simulink library "HORTISIM"  (R2021a)
settings: Solver=VariableStepAuto  StartTime=0.0  StopTime=10.0  RelTol=1e-3
undefined symbols (not defined in the file or in its folder): crop_params, heat_ic, heat_p, p_climate, params_fruit, scr_p, substrate_params, tp_tilapia, win_p, x0_climate, x0_crop, x0_fruit, x0_substrate, x0_tank_tilapia
libraries: $bdroot x10
(part 2 of 4)

== system HORTISIM/Climate/Models/Climate Model/Gases Exchange ==
  Indoor Temperature : Inport
  Transpiration Heat : Inport  Port=2
  Ventilation Rate : Inport  Port=3
  Condensation : Inport  Port=4
  In Bus Element : Inport  Port=5  PortName=EC  Element=Temp
  In Bus Element1 : Inport  Port=5  PortName=EC  Element=HR
  Carbon Consumption : Inport  Port=6
  CO2 Pump : Inport  Port=7
  Carbon Dynamics : Subsystem
      settings: PortSchema="{\"entries\":[{\"content\":{\"sides\":[{\"content\":{\"connectorIds\":[\"In1\",\"In2\",\"In3\"]},\"type\":\"ConnectorPlacement.EquallySpacedRectSide\",\"uuid\":\"ce6da3e3-21f1-4394-8848-c3b9ed37cfe4\"},{\"content\":{\"connectorIds\":[\"Out1\",\"Out2\"],\"side\":\"RIGHT\"},\"type\":\"ConnectorPlacement.EquallySpacedRectSide\",\"uuid\":\"ff9d1dc7-ad1d-4f02-8424-55a857bc099f\"},{\"content\":{\"connectorIds\":[\"In4\",\"In5\"],\"side\":\"TOP\"},\"type\":\"ConnectorPlacement.EquallySpacedRectSide\",\"uuid\":\"728a06d8-4ce2-49f0-80dc-b6302b266d7a\"}]},\"type\":\"ConnectorPlacement.EquallySpacedConnector\",\"uuid\":\"a07ea8b7-add0-4d37-8d5e-856da5f5b640\"}],\"packageUris\":[\"http://schema.mathworks.com/mf0/Connector/R2020b\"],\"version\":\"1.0\"}"
  Compute Mid Variables : Subsystem
      settings: PortSchema="{\"entries\":[{\"content\":{\"sides\":[{\"content\":{\"connectorIds\":[\"In1\",\"In2\"]},\"type\":\"ConnectorPlacement.EquallySpacedRectSide\",\"uuid\":\"c9e251e2-f19d-4856-b15c-3b9f1eb64f83\"},{\"content\":{\"connectorIds\":[\"Out1\"],\"side\":\"RIGHT\"},\"type\":\"ConnectorPlacement.EquallySpacedRectSide\",\"uuid\":\"10734817-c937-42fb-8ae5-9505620c6f0f\"},{\"content\":{\"connectorIds\":[],\"side\":\"TOP\"},\"type\":\"ConnectorPlacement.EquallySpacedRectSide\",\"uuid\":\"8c056440-d8bf-4ff4-85aa-0f6a5eb7f23f\"},{\"content\":{\"connectorIds\":[\"In3\"],\"side\":\"BOTTOM\"},\"type\":\"ConnectorPlacement.EquallySpacedRectSide\",\"uuid\":\"fc2511c5-58d6-455e-9438-4abf6bda86a2\"}]},\"type\":\"ConnectorPlacement.EquallySpacedConnector\",\"uuid\":\"13e72cfa-9d8f-4756-adac-f24fb0238c2a\"}],\"packageUris\":[\"http://schema.mathworks.com/mf0/Connector/R2020b\"],\"version\":\"1.0\"}"
  Gain1 : Gain  Gain=24*3600
  Integrator1 : Integrator  InitialCondition=x0.G0  AbsoluteTolerance=1e-5
  Vector Concatenate : Concatenate
  Water Dynamics : Subsystem
      settings: PortSchema="{\"entries\":[{\"content\":{\"sides\":[{\"content\":{\"connectorIds\":[\"In1\",\"In2\",\"In3\"]},\"type\":\"ConnectorPlacement.EquallySpacedRectSide\",\"uuid\":\"ce6da3e3-21f1-4394-8848-c3b9ed37cfe4\"},{\"content\":{\"connectorIds\":[\"Out1\"],\"side\":\"RIGHT\"},\"type\":\"ConnectorPlacement.EquallySpacedRectSide\",\"uuid\":\"ff9d1dc7-ad1d-4f02-8424-55a857bc099f\"},{\"content\":{\"connectorIds\":[\"In4\"],\"side\":\"TOP\"},\"type\":\"ConnectorPlacement.EquallySpacedRectSide\",\"uuid\":\"728a06d8-4ce2-49f0-80dc-b6302b266d7a\"},{\"content\":{\"connectorIds\":[\"In5\",\"In6\"],\"side\":\"BOTTOM\"},\"type\":\"ConnectorPlacement.EquallySpacedRectSide\",\"uuid\":\"cc1d9c53-b6c6-41b0-b878-c109c9de6d5f\"}]},\"type\":\"ConnectorPlacement.EquallySpacedConnector\",\"uuid\":\"a07ea8b7-add0-4d37-8d5e-856da5f5b640\"}],\"packageUris\":[\"http://schema.mathworks.com/mf0/Connector/R2020b\"],\"version\":\"1.0\"}"
  " Gas" : Outport
  wires:
  Gain1/1 -> Integrator1/1
  Vector Concatenate/1 -> Gain1/1
  Integrator1/1 -> Compute Mid Variables/1(Gas_Conc)
  Transpiration Heat/1 -> Water Dynamics/2(Latent Heat)
  Water Dynamics/1(dC_w_dt) -> Vector Concatenate/1
  Carbon Consumption/1 -> Carbon Dynamics/1(CarbonC)
  Carbon Dynamics/1(dC_c_dt) -> Vector Concatenate/2
  Ventilation Rate/1 -> Carbon Dynamics/5(Ventilation Rate), Water Dynamics/6(Ventilation Rate)
  Indoor Temperature/1 -> Compute Mid Variables/2(Indoor Temperature)
  Compute Mid Variables/1(Gas) -> Water Dynamics/1(GasComp), Carbon Dynamics/3(GasComp), " Gas"/1
  Condensation/1 -> Water Dynamics/3(Condensation)
  CO2 Pump/1 -> Carbon Dynamics/2(MC_cc_i)
  In Bus Element/1 -> Carbon Dynamics/4(Te), Water Dynamics/5(Te)
  In Bus Element1/1 -> Water Dynamics/4(He)
  Carbon Dynamics/2(C_ce) -> Compute Mid Variables/3(C_ce)

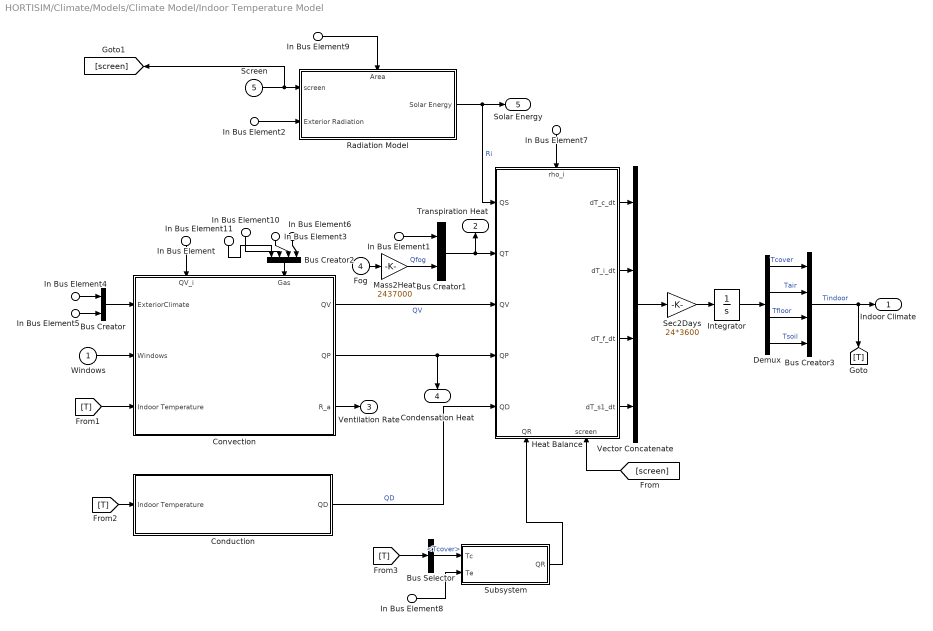
== system HORTISIM/Climate/Models/Climate Model/Indoor Temperature Model ==
  Windows : Inport
  In Bus Element2 : Inport  Port=2  PortName=EC  Element=Rad
  In Bus Element4 : Inport  Port=2  PortName=EC  Element=Temp
  In Bus Element8 : Inport  Port=2  PortName=EC  Element=Temp
  In Bus Element5 : Inport  Port=2  PortName=EC  Element=Wind
  In Bus Element : Inport  Port=3  PortName=External  Element=QV
  In Bus Element1 : Inport  Port=3  PortName=External  Element=QT
  In Bus Element9 : Inport  Port=3  PortName=External  Element=A
  Fog : Inport  Port=4
  Screen : Inport  Port=5
  In Bus Element3 : Inport  Port=6  PortName=Gas  Element=C_w
  In Bus Element6 : Inport  Port=6  PortName=Gas  Element=rho_i
  In Bus Element7 : Inport  Port=6  PortName=Gas  Element=rho_i
  In Bus Element10 : Inport  Port=6  PortName=Gas  Element=C_w_sat_T_c
  In Bus Element11 : Inport  Port=6  PortName=Gas  Element=C_w_sat_T_f
  Bus Creator : BusCreator  Inputs=2
  Bus Creator1 : BusCreator  Inputs=2
  Bus Creator2 : BusCreator  Inputs=4
  Bus Creator3 : BusCreator  Inputs=4
  Bus Selector : BusSelector  OutputSignals=Tcover
  Conduction : Subsystem
  Convection : Subsystem
      settings: PortSchema="{\"entries\":[{\"content\":{\"sides\":[{\"content\":{\"connectorIds\":[\"In1\",\"In2\",\"In3\"]},\"type\":\"ConnectorPlacement.EquallySpacedRectSide\",\"uuid\":\"3a7e199a-659d-4634-89e1-ef85cb7ed502\"},{\"content\":{\"connectorIds\":[\"Out1\",\"Out2\",\"Out3\"],\"side\":\"RIGHT\"},\"type\":\"ConnectorPlacement.EquallySpacedRectSide\",\"uuid\":\"10ed7806-8be5-4e88-a0ca-6abfb5c9ab8d\"},{\"content\":{\"connectorIds\":[\"In4\",\"In5\"],\"side\":\"TOP\"},\"type\":\"ConnectorPlacement.EquallySpacedRectSide\",\"uuid\":\"907defe4-ff8f-4a74-ba27-620529c27b74\"},{\"content\":{\"connectorIds\":[],\"side\":\"BOTTOM\"},\"type\":\"ConnectorPlacement.EquallySpacedRectSide\",\"uuid\":\"397bdb42-e8ee-4be9-8569-3130f6cbf999\"}]},\"type\":\"ConnectorPlacement.EquallySpacedConnector\",\"uuid\":\"f437f85f-61b6-4f41-a544-29e333cf1086\"}],\"packageUris\":[\"http://schema.mathworks.com/mf0/Connector/R2020b\"],\"version\":\"1.0\"}"
  Demux : Demux
  Heat Balance : Subsystem
      settings: PortSchema="{\"entries\":[{\"content\":{\"sides\":[{\"content\":{\"connectorIds\":[\"In1\",\"In2\",\"In3\",\"In4\",\"In5\"]},\"type\":\"ConnectorPlacement.EquallySpacedRectSide\",\"uuid\":\"ccfbb954-e9e7-4841-9dc1-a760315eb250\"},{\"content\":{\"connectorIds\":[\"Out1\",\"Out2\",\"Out3\",\"Out4\"],\"side\":\"RIGHT\"},\"type\":\"ConnectorPlacement.EquallySpacedRectSide\",\"uuid\":\"e9754eb2-54ce-43cf-bf33-7cf2f1345c42\"},{\"content\":{\"connectorIds\":[\"In6\"],\"side\":\"TOP\"},\"type\":\"ConnectorPlacement.EquallySpacedRectSide\",\"uuid\":\"6ccd5de1-b6bb-47c5-ac6c-9382e354fee6\"},{\"content\":{\"connectorIds\":[\"In7\",\"In8\"],\"side\":\"BOTTOM\"},\"type\":\"ConnectorPlacement.EquallySpacedRectSide\",\"uuid\":\"dba41702-708c-4231-8998-8d54661f4881\"}]},\"type\":\"ConnectorPlacement.EquallySpacedConnector\",\"uuid\":\"31920c9d-5e0f-4503-9ddd-ce99d792a3e0\"}],\"packageUris\":[\"http://schema.mathworks.com/mf0/Connector/R2020b\"],\"version\":\"1.0\"}"
  Integrator : Integrator  InitialCondition=x0.T0  AbsoluteTolerance=0.01
  Mass2Heat : Gain  Gain=2437000
  Radiation Model : Subsystem
      settings: PortSchema="{\"entries\":[{\"content\":{\"sides\":[{\"content\":{\"connectorIds\":[\"In1\",\"In2\"]},\"type\":\"ConnectorPlacement.EquallySpacedRectSide\",\"uuid\":\"cb5a2538-07d5-409a-bc47-ac7157db0ef4\"},{\"content\":{\"connectorIds\":[\"Out1\"],\"side\":\"RIGHT\"},\"type\":\"ConnectorPlacement.EquallySpacedRectSide\",\"uuid\":\"7dfe2e6f-8ee6-45c0-8502-080571e1b483\"},{\"content\":{\"connectorIds\":[\"In3\"],\"side\":\"TOP\"},\"type\":\"ConnectorPlacement.EquallySpacedRectSide\",\"uuid\":\"52df64bb-9cf1-44e4-8c24-fa6c372d73f1\"}]},\"type\":\"ConnectorPlacement.EquallySpacedConnector\",\"uuid\":\"b803895f-b114-4368-b273-36a7794022b5\"}],\"packageUris\":[\"http://schema.mathworks.com/mf0/Connector/R2020b\"],\"version\":\"1.0\"}"
  Sec2Days : Gain  Gain=24*3600
  Subsystem : Subsystem
  Vector Concatenate : Concatenate  NumInputs=4
  Indoor Climate : Outport
  Transpiration Heat : Outport  Port=2
  Ventilation Rate : Outport  Port=3
  Condensation Heat : Outport  Port=4
  Solar Energy : Outport  Port=5
  wires:
  [screen] -> Heat Balance/8(screen)
  Vector Concatenate/1 -> Sec2Days/1
  Sec2Days/1 -> Integrator/1
  Convection/3(R_a) -> Ventilation Rate/1
  Convection/1(QV) -> Heat Balance/3(QV)  "QV"
  Conduction/1(QD) -> Heat Balance/5(QD)  "QD"
  Heat Balance/2(dT_i_dt) -> Vector Concatenate/2
  Heat Balance/3(dT_f_dt) -> Vector Concatenate/3
  Heat Balance/4(dT_s1_dt) -> Vector Concatenate/4
  Heat Balance/1(dT_c_dt) -> Vector Concatenate/1
  [T] -> Convection/3(Indoor Temperature)
  [T] -> Conduction/1(Indoor Temperature)
  In Bus Element7/1 -> Heat Balance/6(rho_i)
  Convection/2(QP) -> Condensation Heat/1, Heat Balance/4(QP)
  Windows/1 -> Convection/2(Windows)
  In Bus Element2/1 -> Radiation Model/2(Exterior Radiation)
  Radiation Model/1("Solar Energy  ") -> Solar Energy/1, Heat Balance/1(QS)  "Ri"
  Bus Creator/1 -> Convection/1(ExteriorClimate)
  Screen/1 -> Radiation Model/1(screen), [screen]
  In Bus Element4/1 -> Bus Creator/1
  In Bus Element5/1 -> Bus Creator/2
  Fog/1 -> Mass2Heat/1
  Mass2Heat/1 -> Bus Creator1/2  "Qfog"
  In Bus Element1/1 -> Bus Creator1/1
  Bus Creator1/1 -> Heat Balance/2(QT), Transpiration Heat/1
  Bus Creator2/1 -> Convection/5(Gas)
  In Bus Element3/1 -> Bus Creator2/3
  In Bus Element6/1 -> Bus Creator2/4
  In Bus Element/1 -> Convection/4(QV_i)
  Bus Creator3/1 -> [T], Indoor Climate/1  "Tindoor"
  Demux/4 -> Bus Creator3/4  "Tsoil"
  Demux/3 -> Bus Creator3/3  "Tfloor"
  Demux/2 -> Bus Creator3/2  "Tair"
  Demux/1 -> Bus Creator3/1  "Tcover"
  Integrator/1 -> Demux/1
  In Bus Element8/1 -> Subsystem/2(Te)
  [T] -> Bus Selector/1
  Bus Selector/1 -> Subsystem/1(Tc)  "<Tcover>"
  Subsystem/1(QR) -> Heat Balance/7(QR)
  In Bus Element9/1 -> Radiation Model/3(Area)
  In Bus Element10/1 -> Bus Creator2/2
  In Bus Element11/1 -> Bus Creator2/1

== system HORTISIM/Climate/Models/Climate Model/Subsystem ==
  Gas : Inport
  Bus Creator3 : BusCreator  Inputs=4
  Bus Selector : BusSelector  OutputSignals=C_w,rho_i,C_w_sat_T_c,C_w_sat_T_f
  Out1 : Outport
  wires:
  Bus Selector/3 -> Bus Creator3/3  "<C_w_sat_T_c>"
  Bus Creator3/1 -> Out1/1
  Bus Selector/1 -> Bus Creator3/1  "<C_w>"
  Bus Selector/2 -> Bus Creator3/2  "<rho_i>"
  Bus Selector/4 -> Bus Creator3/4  "<C_w_sat_T_f>"
  Gas/1 -> Bus Selector/1

== system HORTISIM/Horticulture/Controls/Ferrtirrigation Controler/Irrigation Controler ==
  note: $kg\{H_2O\}/(s\cdot m^2)$
  " " : Gain  Gain=5.6e-3
  Clock2 : Clock
  Constant1 : Constant  Value=24
  Gain4 : Gain  Gain=24
  If : If  IfExpression=(u1 > 6)&(u1<7)
  If Action Subsystem : Subsystem  TreatAsAtomicUnit=on
  If Action Subsystem1 : Subsystem  TreatAsAtomicUnit=on
  Merge : Merge
  Mod : Math  Operator=mod  SaturateOnIntegerOverflow=on
  Irrigation : Outport
  wires:
  " "/1 -> Irrigation/1
  Constant1/1 -> Mod/2
  Clock2/1 -> Gain4/1
  Gain4/1 -> Mod/1
  Mod/1 -> If/1, If Action Subsystem/1(In1)
  If/1 -> If Action Subsystem/Action
  If/2 -> If Action Subsystem1/Action
  If Action Subsystem/1(Out1) -> Merge/1
  If Action Subsystem1/1(Out1) -> Merge/2
  Merge/1 -> " "/1

== system HORTISIM/Horticulture/Models/Crop Grow/Air Convection ==
  QS_v_VIS : Inport
  QT_v_i : Inport  Port=2
  T_i : Inport  Port=3
  <LAI> : Inport  Port=4
  " Temperature" : MATLAB Function  TreatAsAtomicUnit=on
  Bus Creator : BusCreator  Inputs=5
  Constant : Constant  Value=params.A_v
  Gain1 : Gain  Gain=24*3600
  Minus : Sum  Inputs=+-
  Subsystem : Subsystem
      settings: PortSchema="{\"entries\":[{\"content\":{\"sides\":[{\"content\":{\"connectorIds\":[\"In1\",\"In2\"]},\"type\":\"ConnectorPlacement.EquallySpacedRectSide\",\"uuid\":\"4a223777-4148-4e71-aff8-25d93471e208\"},{\"content\":{\"connectorIds\":[\"Out1\",\"Out2\"],\"side\":\"RIGHT\"},\"type\":\"ConnectorPlacement.EquallySpacedRectSide\",\"uuid\":\"f67a472e-d82a-4194-8a1d-cf4d17d79652\"},{\"content\":{\"connectorIds\":[],\"side\":\"TOP\"},\"type\":\"ConnectorPlacement.EquallySpacedRectSide\",\"uuid\":\"dc13fded-a670-4e66-896d-6b985aeea447\"},{\"content\":{\"connectorIds\":[\"In3\"],\"side\":\"BOTTOM\"},\"type\":\"ConnectorPlacement.EquallySpacedRectSide\",\"uuid\":\"546dc1d6-9e48-4e4a-b9dc-c8e8ff8af02b\"}]},\"type\":\"ConnectorPlacement.EquallySpacedConnector\",\"uuid\":\"dd1fea49-cd8b-49b4-879c-c05a742382b3\"}],\"packageUris\":[\"http://schema.mathworks.com/mf0/Connector/R2020b\"],\"version\":\"1.0\"}"
  Tv : Integrator  InitialCondition=x0.Tv  AbsoluteTolerance=0.01
  Tv_mean : Integrator  InitialCondition=x0.Tv  AbsoluteTolerance=1e-3
  surface density [kg/m^2] : Constant  Value=1.326
  HV : Outport
  HeatVars : Outport  Port=2
  wires:
  Gain1/1 -> Tv/1
  " Temperature"/1(dT_v_dt) -> Gain1/1
  surface density [kg/m^2]/1 -> " Temperature"/6(msd_v)
  Constant/1 -> " Temperature"/4(A_v)
  <LAI>/1 -> Subsystem/2(LAI), " Temperature"/5(LAI)
  Subsystem/2(HV) -> HV/1
  T_i/1 -> Subsystem/1(T_i)
  Tv_mean/1 -> [Tv_mu], Minus/2  "Tv_mean"
  Minus/1 -> Tv_mean/1
  Tv/1 -> [Tv], Minus/1, Subsystem/3(T_v)  "Tv"
  Subsystem/1(QV_v_i) -> [QV_v_i], " Temperature"/3(QV_v_i)  "QV"
  QS_v_VIS/1 -> [QS_i]  "QS"
  QT_v_i/1 -> [QT_v_i], " Temperature"/2(QT_v_i)  "QT"
  [Tv] -> Bus Creator/1  "Tveg"
  [Tv_mu] -> Bus Creator/2  "TvegMean"
  [QV_v_i] -> Bus Creator/3
  [QT_v_i] -> Bus Creator/4
  [QS_i] -> Bus Creator/5
  Bus Creator/1 -> HeatVars/1

== system HORTISIM/Horticulture/Models/Crop Grow/Crop Growth ==
  Gas : Inport
  QS_v_VIS : Inport  Port=2
  MC_leaf_prune : Inport  Port=3
  harvest : Inport  Port=4
  RTU : Inport  Port=5
  CropBus : Inport  Port=6
  Temperature : Inport  Port=7
  Bus Creator : BusCreator  Inputs=5
  Gain{1..4} (4 alike) : Gain  Gain=24*3600
  Growth model : Subsystem
      settings: PortSchema="{\"entries\":[{\"content\":{\"sides\":[{\"content\":{\"connectorIds\":[\"In1\",\"In2\",\"In3\",\"In4\",\"In5\"]},\"type\":\"ConnectorPlacement.EquallySpacedRectSide\",\"uuid\":\"524d3e03-5719-41db-bf49-dcf5dd5869ab\"},{\"content\":{\"connectorIds\":[\"Out1\",\"Out2\",\"Out3\",\"Out4\",\"Out5\"],\"side\":\"RIGHT\"},\"type\":\"ConnectorPlacement.EquallySpacedRectSide\",\"uuid\":\"b6ee0c40-6a76-4355-a893-3d13d29f29ea\"},{\"content\":{\"connectorIds\":[\"In6\",\"Out6\"],\"side\":\"TOP\"},\"type\":\"ConnectorPlacement.EquallySpacedRectSide\",\"uuid\":\"3cb45a24-0889-4a9a-ac04-e1ca208b77ae\"}]},\"type\":\"ConnectorPlacement.EquallySpacedConnector\",\"uuid\":\"fab17374-053c-4d8a-b11b-d7cd69978ad8\"}],\"packageUris\":[\"http://schema.mathworks.com/mf0/Connector/R2020b\"],\"version\":\"1.0\"}"
  Integrator1 : Integrator  InitialCondition=x0.N  AbsoluteTolerance=1e-4
  Integrator2 : Integrator  InitialCondition=x0.C  AbsoluteTolerance=1e-4
  Integrator3 : Integrator  InitialCondition=x0.R  AbsoluteTolerance=1e-9
  Integrator4 : Integrator  InitialCondition=x0.Tsum
  Subsystem : Subsystem
  Subsystem1 : Subsystem
  Subsystem2 : Subsystem
      settings: PortSchema="{\"entries\":[{\"content\":{\"sides\":[{\"content\":{\"connectorIds\":[\"In1\"]},\"type\":\"ConnectorPlacement.EquallySpacedRectSide\",\"uuid\":\"1f0226fa-6d14-4434-a5d5-098a94c6aa33\"},{\"content\":{\"connectorIds\":[\"Out1\"],\"side\":\"RIGHT\"},\"type\":\"ConnectorPlacement.EquallySpacedRectSide\",\"uuid\":\"12e08114-9d71-45f9-bd21-e03815fbba92\"},{\"content\":{\"connectorIds\":[],\"side\":\"TOP\"},\"type\":\"ConnectorPlacement.EquallySpacedRectSide\",\"uuid\":\"f70b570c-09d2-427a-8272-34c6eabee9a4\"},{\"content\":{\"connectorIds\":[\"In2\"],\"side\":\"BOTTOM\"},\"type\":\"ConnectorPlacement.EquallySpacedRectSide\",\"uuid\":\"db0772f6-92fe-46fe-85e5-ff48d92542ad\"}]},\"type\":\"ConnectorPlacement.EquallySpacedConnector\",\"uuid\":\"23ce1bc9-4d09-4c56-8e1c-5e49b0ef0462\"}],\"packageUris\":[\"http://schema.mathworks.com/mf0/Connector/R2020b\"],\"version\":\"1.0\"}"
  "Carbon Comp   " : Outport
  Crop : Outport  Port=2
  wires:
  Bus Creator/1 -> Crop/1  "Crop"
  Growth model/6("Carbon Comp   ") -> "Carbon Comp   "/1
  MC_leaf_prune/1 -> Growth model/3(MC_leaf_prune)
  Integrator4/1 -> Bus Creator/4  "Tsum"
  Growth model/3(dRdt) -> Gain3/1
  Gas/1 -> Growth model/1(Gas)
  Gain3/1 -> Integrator3/1
  Gain4/1 -> Integrator4/1
  Growth model/4(dT_vsum_dt) -> Gain4/1
  Growth model/2(dCdt) -> Gain2/1
  QS_v_VIS/1 -> Growth model/2(QS_v_VIS)
  Gain2/1 -> Integrator2/1
  CropBus/1 -> Growth model/4(Crop)
  Temperature/1 -> Growth model/5(Temperature)
  Growth model/5(MC_gro) -> Bus Creator/5  "MC_gro"
  Subsystem/1(Out1) -> Bus Creator/2  "Carbon"
  Integrator2/1 -> Subsystem/1(In1)  "Carbon"
  Integrator3/1 -> Subsystem1/1(In1)  "Relative"
  Subsystem1/1(Out1) -> Bus Creator/3  "Relative"
  Gain1/1 -> Integrator1/1
  RTU/1 -> Gain1/1  "Nuptake"
  Integrator1/1 -> Subsystem2/1(M)  "Nutrients"
  Subsystem2/1(Out1) -> Bus Creator/1  "Nutrients"
  Growth model/1(dN/dt) -> Subsystem2/2(ND)  "Ndemand"
  harvest/1 -> Growth model/6(harvest)

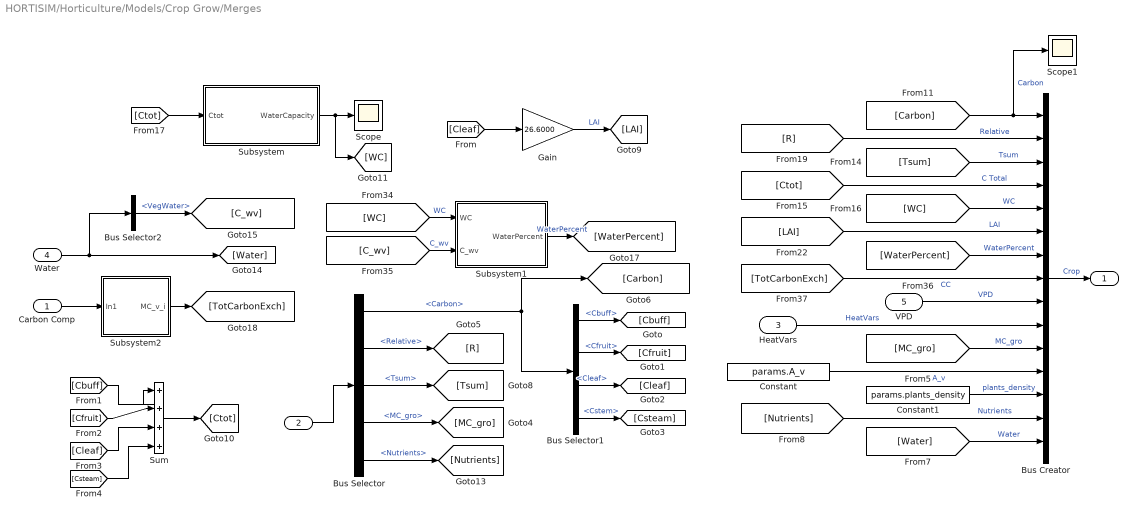
== system HORTISIM/Horticulture/Models/Crop Grow/Merges ==
  "Carbon Comp   " : Inport
  " " : Inport  Port=2
  HeatVars : Inport  Port=3
  Water : Inport  Port=4
  VPD : Inport  Port=5
  Bus Creator : BusCreator  Inputs=15
  Bus Selector : BusSelector  OutputSignals=Carbon,Relative,Tsum,MC_gro,Nutrients
  Bus Selector1 : BusSelector  OutputSignals=Cbuff,Cfruit,Cleaf,Cstem
  Bus Selector2 : BusSelector  OutputSignals=WaterState.VegWater
  Constant : Constant  Value=params.A_v
  Constant1 : Constant  Value=params.plants_density
  Gain : Gain  Gain=26.6000
  Scope : Scope
  Scope1 : Scope
  Subsystem : Subsystem
  Subsystem1 : Subsystem
  Subsystem2 : Subsystem
  Sum : Sum  Inputs=|++++
  "    " : Outport
  wires:
  [Cleaf] -> Gain/1
  Gain/1 -> [LAI]  "LAI"
  Subsystem/1(WaterCapacity) -> [WC], Scope/1
  [Ctot] -> Subsystem/1(Ctot)
  [Cbuff] -> Sum/1
  [Cfruit] -> Sum/2
  [Cleaf] -> Sum/3
  Sum/1 -> [Ctot]
  Bus Selector/1 -> Bus Selector1/1, [Carbon]  "<Carbon>"
  Water/1 -> Bus Selector2/1, [Water]
  [Tsum] -> Bus Creator/3  "Tsum"
  [LAI] -> Bus Creator/6  "LAI"
  [R] -> Bus Creator/2  "Relative"
  " "/1 -> Bus Selector/1
  Bus Selector1/1 -> [Cbuff]  "<Cbuff>"
  Bus Selector1/3 -> [Cleaf]  "<Cleaf>"
  Bus Creator/1 -> "    "/1  "Crop"
  Bus Selector1/4 -> [Csteam]  "<Cstem>"
  [WC] -> Subsystem1/1(WC)  "WC"
  Subsystem1/1(WaterPercent) -> [WaterPercent]  "WaterPercent"
  [TotCarbonExch] -> Bus Creator/8  "CC"
  VPD/1 -> Bus Creator/9  "VPD"
  [WC] -> Bus Creator/5  "WC"
  Bus Selector/4 -> [MC_gro]  "<MC_gro>"
  [MC_gro] -> Bus Creator/11  "MC_gro"
  HeatVars/1 -> Bus Creator/10  "HeatVars"
  [Csteam] -> Sum/4
  Constant/1 -> Bus Creator/12  "A_v"
  [WaterPercent] -> Bus Creator/7  "WaterPercent"
  [Water] -> Bus Creator/15  "Water"
  [Carbon] -> Scope1/1, Bus Creator/1  "Carbon"
  Bus Selector/3 -> [Tsum]  "<Tsum>"
  "Carbon Comp   "/1 -> Subsystem2/1(In1)
  Bus Selector1/2 -> [Cfruit]  "<Cfruit>"
  Bus Selector/2 -> [R]  "<Relative>"
  Bus Selector2/1 -> [C_wv]  "<VegWater>"
  [C_wv] -> Subsystem1/2(C_wv)  "C_wv"
  Subsystem2/1(MC_v_i) -> [TotCarbonExch]
  [Ctot] -> Bus Creator/4  "C Total"
  Constant1/1 -> Bus Creator/13  "plants_density"
  Bus Selector/5 -> [Nutrients]  "<Nutrients>"
  [Nutrients] -> Bus Creator/14  "Nutrients"

== system HORTISIM/Horticulture/Models/Crop Grow/Subsystem ==
  In1 : Inport
  In2 : Inport  Port=2
  In3 : Inport  Port=3
  Bus Selector : BusSelector  OutputSignals=LAI
  Constant1 : Constant  Value=params.A_v
  Gain : Gain  Gain=2
  Product1 : Product  Inputs=3
  Scope : Scope
  Scope1 : Scope
  Subsystem : Subsystem
  Subsystem1 : Subsystem
  Sum : Sum  Inputs=|++
  Sum1 : Sum  Inputs=|++
  Out1 : Outport
  wires:
  In2/1 -> Sum1/2
  Sum1/1 -> Product1/3
  In1/1 -> Sum1/1
  Constant1/1 -> Product1/2
  In3/1 -> Bus Selector/1
  Subsystem/1(Out1) -> Scope/1, [a_v_fVIS]
  Bus Selector/1 -> Subsystem1/1(<LAI>), Subsystem/1(<LAI>)  "<LAI>"
  Subsystem1/1(Out1) -> [a_v_rVIS]
  [a_v_rVIS] -> Sum/1
  [a_v_fVIS] -> Sum/2
  Sum/1 -> Scope1/1, Product1/1
  Product1/1 -> Gain/1
  Gain/1 -> Out1/1

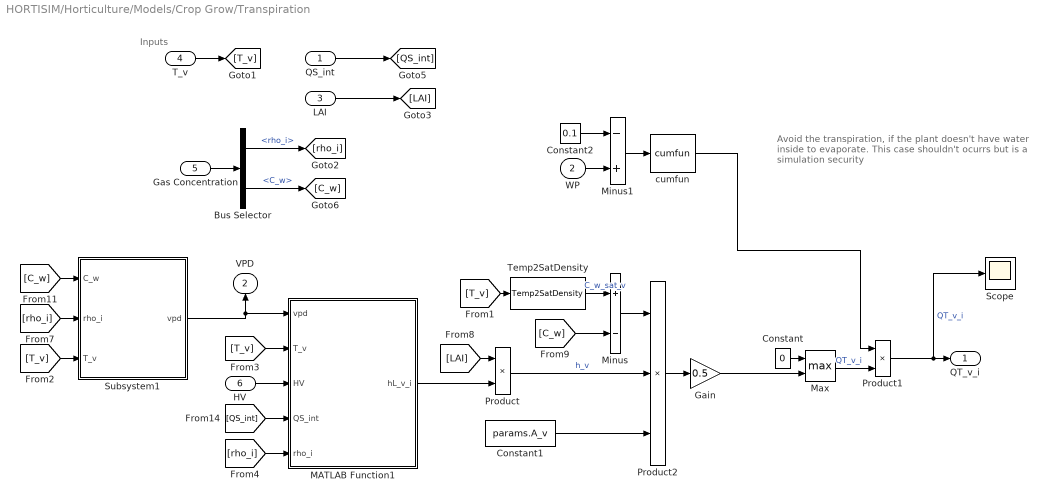
== system HORTISIM/Horticulture/Models/Crop Grow/Transpiration ==
  note: Avoid the transpiration, if the plant
      |  doesn't have water inside to evaporate.
      | This case shouldn't ocurrs but is a simulation security
  note: Inputs
  QS_int : Inport
  WP : Inport  Port=2
  LAI : Inport  Port=3
  T_v : Inport  Port=4
  Gas Concentration : Inport  Port=5
  HV : Inport  Port=6
  Bus Selector : BusSelector  OutputSignals=rho_i,C_w
  Constant : Constant  Value=0
  Constant1 : Constant  Value=params.A_v
  Constant2 : Constant  Value=0.1
  Gain : Gain  Gain=0.5
  MATLAB Function1 : MATLAB Function  TreatAsAtomicUnit=on
  Max : MinMax  Function=max  Inputs=2
  Minus : Sum  Inputs=+-
  Minus1 : Sum  Inputs=-+
  Product : Product
  Product1 : Product
  Product2 : Product  Inputs=3
  Scope : Scope
  Subsystem1 : Subsystem
  Temp2SatDensity : $bdroot/Other  Functions/Temp2SatDensity  SystemSampleTime=-1  VariantActivationTime=update diagram  Latency=0  AutoFrameSizeCalculation=off
  cumfun : $bdroot/Other  Functions/cumfun  SystemSampleTime=-1  VariantActivationTime=update diagram  Latency=0  AutoFrameSizeCalculation=off
  QT_v_i : Outport
  VPD : Outport  Port=2
  wires:
  Gain/1 -> Max/2
  Max/1 -> Product1/2  "QT_v_i"
  Constant/1 -> Max/1
  Product1/1 -> Scope/1, QT_v_i/1  "QT_v_i"
  Product2/1 -> Gain/1
  Constant1/1 -> Product2/3
  Product/1 -> Product2/2  "h_v"
  Minus/1 -> Product2/1
  [C_w] -> Minus/2
  T_v/1 -> [T_v]
  QS_int/1 -> [QS_int]
  Gas Concentration/1 -> Bus Selector/1
  Bus Selector/1 -> [rho_i]  "<rho_i>"
  Bus Selector/2 -> [C_w]  "<C_w>"
  [T_v] -> Temp2SatDensity/1
  Temp2SatDensity/1 -> Minus/1  "C_w_sat_v"
  [C_w] -> Subsystem1/1(C_w)
  [rho_i] -> Subsystem1/2(rho_i)
  [T_v] -> Subsystem1/3(T_v)
  LAI/1 -> [LAI]
  [LAI] -> Product/1
  MATLAB Function1/1(hL_v_i) -> Product/2
  [QS_int] -> MATLAB Function1/4(QS_int)
  HV/1 -> MATLAB Function1/3(HV)
  Subsystem1/1(vpd) -> VPD/1, MATLAB Function1/1(vpd)
  [T_v] -> MATLAB Function1/2(T_v)
  [rho_i] -> MATLAB Function1/5(rho_i)
  WP/1 -> Minus1/2
  Constant2/1 -> Minus1/1
  cumfun/1 -> Product1/1
  Minus1/1 -> cumfun/1

== system HORTISIM/Horticulture/Models/Crop Grow/Water Balance ==
  note: $kg\{H_2O\}/(s\cdot m^2)$
  note: $kg\{H_2O\}/m^2$
  note: $kg\{H_2O\}/(s\cdot m^2)$
  Crop : Inport
  <QT_v_i> : Inport  Port=2
  RWU : Inport  Port=3
  Bus Selector : BusSelector  OutputSignals=WaterPercent,WC,A_v
  Divide : Product  Inputs=*//
  H_fg : Constant  Value=2437000
  Subsystem : Subsystem
  Subsystem1 : Subsystem
  Out Bus Element : Outport  PortName=WaterFlows  Element=WaterDemand
  Out Bus Element1 : Outport  PortName=WaterFlows  Element=WaterUptake
  Out Bus Element3 : Outport  PortName=WaterFlows  Element=MW_QT
  Out Bus Element6 : Outport  Port=2  PortName=WaterState  Element=VegWater
  wires:
  Divide/1 -> [MW_QT], Subsystem/2(Evapotranspiration)  "Evapotranspiration"
  <QT_v_i>/1 -> Divide/1
  H_fg/1 -> Divide/2
  Crop/1 -> Bus Selector/1
  [RWU] -> Out Bus Element1/1  "Real Water Uptake"
  [DemandWater] -> Out Bus Element/1
  Bus Selector/3 -> Divide/3  "<A_v>"
  Bus Selector/1 -> Subsystem1/1(<WaterPercent>)  "<WaterPercent>"
  Bus Selector/2 -> Subsystem1/2(<WC>)  "<WC>"
  Subsystem1/1(Out1) -> [DemandWater]
  RWU/1 -> [RWU], Subsystem/1(Real Water Uptake)  "Real Water Uptake"
  Subsystem/1(C_wv) -> Out Bus Element6/1
  [MW_QT] -> Out Bus Element3/1

== system HORTISIM/Horticulture/Models/Substrate Bag/Nutrient Balance ==
  Irrigation : Inport
  NutrientDemand : Inport  Port=2
  Water : Inport  Port=3
  Bus Creator : BusCreator  Inputs=3  OutDataTypeStr=Bus: FLOW  NonVirtualBus=on
  Bus Selector1 : BusSelector  OutputSignals=X,f,T
  Bus Selector3 : BusSelector  OutputSignals=Water,SusWater.VT,drainge
  Demux : Demux  Outputs=8
  Gain1 : Gain  Gain=24*3600
  Integrator : Integrator  InitialCondition=x0.N
  Minus : Sum  Inputs=-+--
  Product : Product
  Product2 : Product
  Product3 : Product
  Scope : Scope
  Subsystem : Subsystem
  Subsystem1 : Subsystem
  Vector Concatenate : Concatenate  NumInputs=8
  Drainge : Outport
  Mass In Sustrate : Outport  Port=2
  RealNutrientUptake : Outport  Port=3
  wires:
  Irrigation/1 -> Bus Selector1/1  "Irrigation"
  Bus Selector1/1 -> Product/1  "<X>"
  Bus Selector1/2 -> Product/2  "<f>"
  Product/1 -> Demux/1
  Integrator/1 -> Scope/1, Subsystem/2(Mass), Mass In Sustrate/1, Subsystem1/2(Content)
  Product2/1 -> Minus/4
  Bus Selector1/3 -> [T]  "<T>"
  [T] -> Bus Creator/2  "T"
  [D] -> Bus Creator/1  "f"
  Bus Creator/1 -> Drainge/1
  Subsystem/1(X) -> Product3/2, Product2/1, Bus Creator/3
  Vector Concatenate/1 -> Minus/2
  Minus/1 -> Gain1/1
  Gain1/1 -> Integrator/1
  NutrientDemand/1 -> Subsystem1/1(Demand)
  Subsystem1/1(RealNutrientUptake) -> Minus/1, RealNutrientUptake/1
  Water/1 -> Bus Selector3/1
  Bus Selector3/1 -> [WPT]  "<Water>"
  Bus Selector3/2 -> [SW]  "<VT>"
  Bus Selector3/3 -> [D]  "<drainge>"
  [D] -> Product2/2
  [SW] -> Subsystem/1(V)
  [WPT] -> Product3/1
  Product3/1 -> Minus/3
  Demux/8 -> Vector Concatenate/8  "TSS"
  Demux/7 -> Vector Concatenate/7  "O2"
  Demux/6 -> Vector Concatenate/6  "S"
  Demux/5 -> Vector Concatenate/5  "P"
  Demux/4 -> Vector Concatenate/4  "Mg"
  Demux/3 -> Vector Concatenate/3  "Ca"
  Demux/2 -> Vector Concatenate/2  "K"
  Demux/1 -> Vector Concatenate/1  "N"

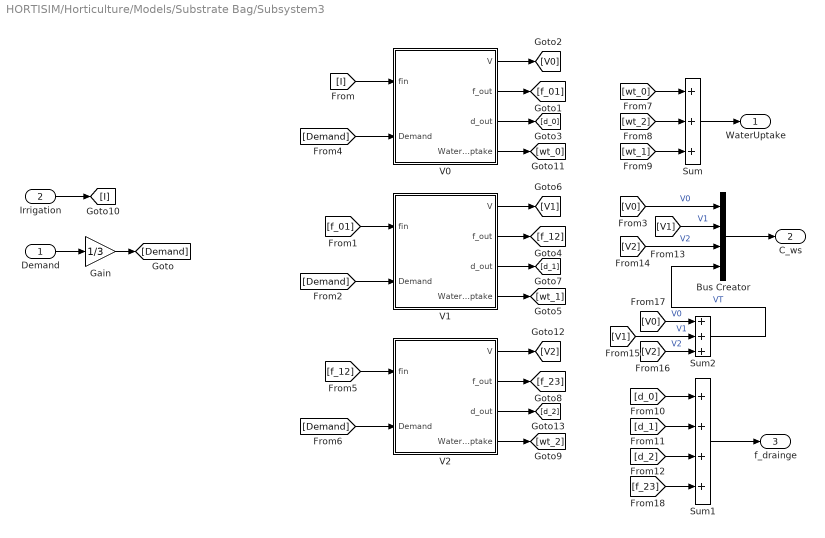
== system HORTISIM/Horticulture/Models/Substrate Bag/Subsystem3 ==
  Demand : Inport
  Irrigation : Inport  Port=2
  Bus Creator : BusCreator  Inputs=4
  Gain : Gain  Gain=1/3
  Sum : Sum  Inputs=+++
  Sum1 : Sum  Inputs=++++
  Sum2 : Sum  Inputs=+++
  V0 : Subsystem
  V1 : Subsystem
  V2 : Subsystem
  WaterUptake : Outport
  C_ws : Outport  Port=2
  f_drainge : Outport  Port=3
  wires:
  [I] -> V0/1(fin)
  V0/1(V) -> [V0]
  V0/2(f_out) -> [f_01]
  V0/3(d_out) -> [d_0]
  Irrigation/1 -> [I]
  Sum1/1 -> f_drainge/1
  Demand/1 -> Gain/1
  Gain/1 -> [Demand]
  [Demand] -> V0/2(Demand)
  V0/4(WaterUptake) -> [wt_0]
  V1/3(d_out) -> [d_1]
  V1/4(WaterUptake) -> [wt_1]
  V1/2(f_out) -> [f_12]
  [Demand] -> V1/2(Demand)
  V1/1(V) -> [V1]
  [f_12] -> V2/1(fin)
  V2/3(d_out) -> [d_2]
  V2/4(WaterUptake) -> [wt_2]
  V2/2(f_out) -> [f_23]
  [Demand] -> V2/2(Demand)
  V2/1(V) -> [V2]
  [f_01] -> V1/1(fin)
  [wt_0] -> Sum/1
  [wt_2] -> Sum/2
  [wt_1] -> Sum/3
  Sum/1 -> WaterUptake/1
  [d_2] -> Sum1/3
  [d_1] -> Sum1/2
  [d_0] -> Sum1/1
  [V0] -> Bus Creator/1  "V0"
  [V1] -> Bus Creator/2  "V1"
  [V2] -> Bus Creator/3  "V2"
  Bus Creator/1 -> C_ws/1
  [V0] -> Sum2/1  "V0"
  [V1] -> Sum2/2  "V1"
  [V2] -> Sum2/3  "V2"
  Sum2/1 -> Bus Creator/4  "VT"
  [f_23] -> Sum1/4

== system HORTISIM/Aquaculture/Models/Tank Model/Heat Balances/Convection Air 2 Water Tanl Surface ==
  T_i : Inport
  A_t : Inport  Port=2
  T_w : Inport  Port=3
  d_t : Inport  Port=4
  wind_speed : Inport  Port=5
  Divide : Product  Inputs=*/
  Gr : Subsystem
  Gr2vG : Subsystem
  Minus : Sum  Inputs=-+
  Product : Product  Inputs=4
  Re : Subsystem
  Re2vR : Subsystem
  Subsystem : Subsystem
  "thermal conductivity of air [W/m/K] " : Constant  Value=0.0250
  QV_i_w : Outport
  wires:
  T_i/1 -> [T_i]
  T_w/1 -> [T_w]
  A_t/1 -> [A_t]
  d_t/1 -> [d_t]
  wind_speed/1 -> [ws]
  [ws] -> Re/2(wind_speed)
  [d_t] -> Re/1(d_w)
  [T_w] -> Gr/3(T_w)
  [T_i] -> Gr/2(T_air)
  [d_t] -> Gr/1(d)
  Gr/1(Gr) -> Gr2vG/1(Gr)
  Re/1(Re) -> Re2vR/1(Re)
  [A_t] -> Divide/1
  [d_t] -> Divide/2
  Subsystem/1(nu) -> Product/3
  Divide/1 -> Product/2
  "thermal conductivity of air [W/m/K] "/1 -> Product/1
  [T_w] -> Minus/1
  [T_i] -> Minus/2
  Minus/1 -> Product/4
  Product/1 -> QV_i_w/1
  Gr2vG/1(Out1) -> Subsystem/1(In1)
  Gr2vG/2(Out2) -> Subsystem/2(In2)
  Re2vR/1(Out1) -> Subsystem/3(In3)
  Re2vR/2(Out2) -> Subsystem/4(In4)

== system HORTISIM/Aquaculture/Models/Tank Model/Heat Balances/Convection Air 2 Water Tanl Surface1 ==
  T_w : Inport
  A_t : Inport  Port=2
  T_wall : Inport  Port=3
  d_t : Inport  Port=4
  Divide : Product  Inputs=*/
  Minus : Sum  Inputs=+-
  Product : Product  Inputs=3
  "thermal conductivity of air [W/m/K] " : Constant  Value=0.6
  QV_i_w : Outport
  wires:
  T_w/1 -> Minus/2
  T_wall/1 -> Minus/1
  A_t/1 -> Divide/1
  d_t/1 -> Divide/2
  Divide/1 -> Product/2
  "thermal conductivity of air [W/m/K] "/1 -> Product/1
  Minus/1 -> Product/3
  Product/1 -> QV_i_w/1

== system HORTISIM/Aquaculture/Models/Tank Model/Heat Balances/Energy Balance ==
  QV_i_W : Inport
  V : Inport  Port=2
  QA : Inport  Port=3
  QT : Inport  Port=4
  QV_wall_water : Inport  Port=5
  Divide : Product  Inputs=*/
  Integrator1 : Integrator  InitialCondition=x0.T
  J/(kg.K) : Constant  Value=4192
  Product : Product  Inputs=3
  Scope : Scope  NumInputPorts=4
  Sum1 : Sum  Inputs=+-++
  kg/m^3 : Constant  Value=997
  seconds to days1 : Gain  Gain=(3600*24)
  Out1 : Outport
  wires:
  QA/1 -> Sum1/4, Scope/4
  Integrator1/1 -> Out1/1
  Product/1 -> Divide/2  "J/K"
  Sum1/1 -> Divide/1
  seconds to days1/1 -> Integrator1/1
  J/(kg.K)/1 -> Product/2
  kg/m^3/1 -> Product/3
  QV_i_W/1 -> Sum1/3, Scope/3
  Divide/1 -> seconds to days1/1
  V/1 -> Product/1
  QT/1 -> Sum1/2, Scope/2
  QV_wall_water/1 -> Sum1/1, Scope/1

== system HORTISIM/Aquaculture/Models/Tank Model/Heat Balances/Transpiration ==
  Air Speed : Inport
  Xh : Inport  Port=2
  Tw : Inport  Port=3
  p_a : Inport  Port=4
  Constant : Constant  Value=0
  Constant1 : Constant  Value=25
  Constant2 : Constant  Value=params.S
  Divide : Product  Inputs=*/
  Gain : Gain  Gain=19
  Gain1 : Gain  Gain=1/3600
  Mass2Heat [J/kg] : Gain  Gain=2437000
  Max : MinMax  Function=max  Inputs=2
  Minus1 : Sum  Inputs=+-
  Product : Product
  Product1 : Product
  Ratio of Humidity Sat : Subsystem
  Scope : Scope  NumInputPorts=3
  Sum1 : Sum  Inputs=|++
  Water Density [kg/m^3] : Constant  Value=997
  QT : Outport
  Evaporation : Outport  Port=2
  wires:
  Max/1 -> Mass2Heat [J/kg]/1, Divide/1
  Constant/1 -> Max/2
  Divide/1 -> Evaporation/1
  Mass2Heat [J/kg]/1 -> QT/1  "Qfog"
  Water Density [kg/m^3]/1 -> Divide/2
  Product1/1 -> Max/1  "MW_evaporation [kg/s]"
  Product/1 -> Gain1/1
  Constant1/1 -> Sum1/2
  Sum1/1 -> Product/1
  Constant2/1 -> Product/2
  Gain1/1 -> Product1/1
  Air Speed/1 -> Gain/1
  Xh/1 -> Scope/3, Minus1/2
  Gain/1 -> Sum1/1
  Minus1/1 -> Scope/1, Product1/2
  Tw/1 -> Ratio of Humidity Sat/1(T)
  p_a/1 -> Ratio of Humidity Sat/2(p_a)
  Ratio of Humidity Sat/1(Out1) -> Minus1/1, Scope/2  "Xh_sat"

== system HORTISIM/Aquaculture/Models/Tank Model/Subsystem/For Each Subsystem ==
  In1 : Inport  Partition=on  PartitionDimension=1  PartitionWidth=1  PartitionOffset=0
  In2 : Inport  Port=2
  For Each : ForEach  DisableCoverage=on
  Product : Product
  Out1 : Outport  ConcatenationDimension=2
  wires:
  In1/1 -> Product/1
  In2/1 -> Product/2
  Product/1 -> Out1/1

== system HORTISIM/Aquaculture/Models/Tank Model/Subsystem/Subsystem1 ==
  Fio : Inport
  X : Inport  Port=2
  T : Inport  Port=3
  Constant : Constant  Value=0
  For Each Subsystem : Subsystem  TreatAsAtomicUnit=on
  For Each Subsystem1 : Subsystem  TreatAsAtomicUnit=on
  Max : MinMax  Function=max  Inputs=2
  Minus : Sum  Inputs=+-
  Product : Product
  Sum of Elements : Sum  Inputs=+
  Sum of Elements1 : Sum  Inputs=+  CollapseMode=Specified dimension  CollapseDim=2
  Transpose : Math  Operator=transpose  SaturateOnIntegerOverflow=on
  density and specify heat of water : Gain  Gain=997*4186
  fT : Outport
  MS : Outport  Port=2
  QA : Outport  Port=3
  wires:
  Constant/1 -> Max/1
  For Each Subsystem/3(T) -> Minus/1
  Max/1 -> Product/1
  density and specify heat of water/1 -> QA/1
  Minus/1 -> Product/2
  Product/1 -> density and specify heat of water/1
  T/1 -> Minus/2
  Fio/1 -> For Each Subsystem/1(Fin)
  For Each Subsystem/1(fs) -> Sum of Elements/1, Max/2, Transpose/1
  Sum of Elements/1 -> fT/1
  For Each Subsystem/2(Xs) -> For Each Subsystem1/1(fs)
  Transpose/1 -> For Each Subsystem1/2(ps)
  For Each Subsystem1/1(Out1) -> Sum of Elements1/1
  Sum of Elements1/1 -> MS/1
  X/1 -> For Each Subsystem/2(X)

== system HORTISIM/Aquaculture/Models/Tank Model/Subsystem/Subsystem2 ==
  Fin : Inport
  T : Inport  Port=2
  For Each Subsystem : Subsystem  TreatAsAtomicUnit=on
  For Each Subsystem1 : Subsystem  TreatAsAtomicUnit=on
  Minus : Sum  Inputs=+-
  Product : Product
  Sum of Elements : Sum  Inputs=+
  Sum of Elements1 : Sum  Inputs=+  CollapseMode=Specified dimension  CollapseDim=2
  Transpose : Math  Operator=transpose  SaturateOnIntegerOverflow=on
  density and specify heat of water : Gain  Gain=997*4186
  fT : Outport
  MS : Outport  Port=2
  QA : Outport  Port=3
  wires:
  density and specify heat of water/1 -> QA/1
  Product/1 -> density and specify heat of water/1
  Minus/1 -> Product/2
  T/1 -> Minus/2
  For Each Subsystem/3(Ts) -> Minus/1
  Fin/1 -> For Each Subsystem/1(Fin)
  For Each Subsystem/1(fs) -> Transpose/1, Product/1, Sum of Elements/1
  Sum of Elements/1 -> fT/1
  For Each Subsystem/2(Xs) -> For Each Subsystem1/1(fs)
  Transpose/1 -> For Each Subsystem1/2(ps)
  For Each Subsystem1/1(Out1) -> Sum of Elements1/1
  Sum of Elements1/1 -> MS/1

== system HORTISIM/Climate/Controls/Fogging Controler/Subsystem/Subsystem2 ==
  Signal : Inport
  " Min" : Inport  Port=2
  Max : Inport  Port=3
  If : If  NumInputs=3  IfExpression=u2 > u1  ElseIfExpressions=u2 < u3  ZeroCross=off
  If Action Subsystem : Subsystem  TreatAsAtomicUnit=on
  If Action Subsystem1 : Subsystem  TreatAsAtomicUnit=on
  If Action Subsystem2 : Subsystem  TreatAsAtomicUnit=on
  Memory : Memory
  Merge : Merge  Inputs=3
  y : Outport
  wires:
  Signal/1 -> If/2
  " Min"/1 -> If/3
  Max/1 -> If/1
  If/1 -> If Action Subsystem/Action
  If/2 -> If Action Subsystem1/Action
  If/3 -> If Action Subsystem2/Action
  If Action Subsystem2/1(Out1) -> Merge/3
  If Action Subsystem1/1(Out1) -> Merge/2
  If Action Subsystem/1(Out1) -> Merge/1
  Merge/1 -> Memory/1, y/1
  Memory/1 -> If Action Subsystem2/1(In1)

== system HORTISIM/Climate/Controls/Heating Controler/Subsystem/Subsystem1 ==
  Ti : Inport
  A_h_exp : Inport  Port=2
  Th : Inport  Port=3
  Divide2 : Product  Inputs=****/
  Subsystem : Subsystem
  d_h1 : Constant  Value=1.5
  lambda thermal conductivity of air [W/m/K] : Constant  Value=0.025
  QV_h_i : Outport
  wires:
  Ti/1 -> Subsystem/1(Ti)
  Th/1 -> Subsystem/2(Th)
  lambda thermal conductivity of air [W/m/K]/1 -> Divide2/1
  A_h_exp/1 -> Divide2/3
  d_h1/1 -> Divide2/5
  Subsystem/1(Gr) -> Divide2/2
  Subsystem/2(dT) -> Divide2/4
  Divide2/1 -> QV_h_i/1

== system HORTISIM/Climate/Controls/Heating Controler/Subsystem/Subsystem2 ==
  Te : Inport
  A_h_exp : Inport  Port=2
  Th : Inport  Port=3
  Divide2 : Product  Inputs=****/
  Subsystem : Subsystem
  d_h1 : Constant  Value=1.5
  lambda thermal conductivity of air [W/m/K] : Constant  Value=0.025
  QV_h_e : Outport
  wires:
  Te/1 -> Subsystem/1(Ti)
  Th/1 -> Subsystem/2(Th)
  lambda thermal conductivity of air [W/m/K]/1 -> Divide2/1
  A_h_exp/1 -> Divide2/3
  d_h1/1 -> Divide2/5
  Subsystem/1(Gr) -> Divide2/2
  Subsystem/2(dT) -> Divide2/4
  Divide2/1 -> QV_h_e/1

== system HORTISIM/Climate/Controls/Heating Controler/Subsystem2/If Action Subsystem ==
  Action Port : ActionPort
  Constant : Constant  Value=0
  Out1 : Outport
  wires:
  Constant/1 -> Out1/1

== system HORTISIM/Climate/Controls/Heating Controler/Subsystem2/If Action Subsystem1 ==
  Action Port : ActionPort
  Constant : Constant
  Out1 : Outport
  wires:
  Constant/1 -> Out1/1

== system HORTISIM/Climate/Controls/Heating Controler/Subsystem2/If Action Subsystem2 ==
  In1 : Inport
  Action Port : ActionPort
  Out1 : Outport
  wires:
  In1/1 -> Out1/1

== system HORTISIM/Climate/Controls/Screen Controler/Subsystem/If Action Subsystem ==
  Action Port : ActionPort
  Constant : Constant  Value=100
  Out1 : Outport
  wires:
  Constant/1 -> Out1/1

== system HORTISIM/Climate/Controls/Screen Controler/Subsystem/If Action Subsystem1 ==
  EC : Inport
  Action Port : ActionPort
  Constant : Constant  Value=params.Radthreshold
  Gain1 : Gain  Gain=100
  Minus1 : Sum  Inputs=+-
  "Theta " : Subsystem
  Out1 : Outport
  wires:
  Gain1/1 -> Out1/1
  EC/1 -> Minus1/1
  Minus1/1 -> "Theta "/1(In1)
  "Theta "/1(Out1) -> Gain1/1
  Constant/1 -> Minus1/2

== system HORTISIM/Climate/Controls/Screen Controler/Subsystem/Smooth Rad ==
  In1 : Inport
  Integrator1 : Integrator
  Minus2 : Sum  Inputs=+-
  Sec2Days1 : Gain  Gain=24*3600
  Out1 : Outport
  wires:
  Integrator1/1 -> Minus2/2, Out1/1
  Minus2/1 -> Sec2Days1/1
  Sec2Days1/1 -> Integrator1/1
  In1/1 -> Minus2/1

== system HORTISIM/Climate/Models/Climate Model/Gases Exchange/Carbon Dynamics ==
  CarbonC : Inport
  MC_cc_i : Inport  Port=2
  GasComp : Inport  Port=3
  Te : Inport  Port=4
  Ventilation Rate : Inport  Port=5
  Bus Selector1 : BusSelector  OutputSignals=C_c
  Carbon Exchange Indoor-Outdoor : Subsystem
  Constant : Constant  Value=params.V
  Constant1 : Constant  Value=params.V
  Divide : Product  Inputs=/*
  Divide1 : Product  Inputs=*/
  External CO2 Concentration : Subsystem
  Scope : Scope  NumInputPorts=3
  Scope1 : Scope
  Sum1 : Sum  Inputs=|++-
  dC_c_dt : Outport
  C_ce : Outport  Port=2
  wires:
  Ventilation Rate/1 -> Carbon Exchange Indoor-Outdoor/1(R_a)
  CarbonC/1 -> Divide/2
  GasComp/1 -> Bus Selector1/1
  Bus Selector1/1 -> Carbon Exchange Indoor-Outdoor/2(C_c)  "<C_c>"
  External CO2 Concentration/1(C_ce) -> Scope1/1, C_ce/1, Carbon Exchange Indoor-Outdoor/3(C_ce)  "C_ce"
  MC_cc_i/1 -> Divide1/1
  Divide/1 -> Scope/1, Sum1/1  "MC_v_i"
  Divide1/1 -> Scope/2, Sum1/2  "MC_iny"
  Carbon Exchange Indoor-Outdoor/1(MC_i_e) -> Scope/3, Sum1/3  "MC_i_e"
  Sum1/1 -> dC_c_dt/1
  Te/1 -> External CO2 Concentration/1(T_e)
  Constant/1 -> Divide1/2
  Constant1/1 -> Divide/1

== system HORTISIM/Climate/Models/Climate Model/Gases Exchange/Compute Mid Variables ==
  Gas_Conc : Inport
  Indoor Temperature : Inport  Port=2
  C_ce : Inport  Port=3
  Bus Creator : BusCreator  Inputs=12
  Constant : Constant  Value=params.int_air_speed
  Demux : Demux  Outputs=2
  Subsystem : Subsystem
  Gas : Outport
  wires:
  Gas_Conc/1 -> Demux/1, Subsystem/1(Gas_Conc)
  Bus Creator/1 -> Gas/1  "Gas"
  Subsystem/1(rho_i) -> Bus Creator/4  "rho_i"
  Subsystem/2(C_c_ppm) -> Bus Creator/5  "C_c_ppm"
  Subsystem/3(HRInt) -> Bus Creator/6  "HRInt"
  Demux/2 -> Bus Creator/3  "C_c"
  Indoor Temperature/1 -> Subsystem/2(IndoorTemp)
  Constant/1 -> Bus Creator/1  "air_speed"
  Demux/1 -> Bus Creator/2  "C_w"
  Subsystem/6(xH) -> Bus Creator/9  "Xh"
  Subsystem/4(C_w_sat_T_c) -> Bus Creator/7  "C_w_sat_T_c"
  Subsystem/5(C_w_sat_T_f) -> Bus Creator/8  "C_w_sat_T_f"
  Subsystem/7(p_a) -> Bus Creator/10  "p_a"
  Subsystem/8(xH_sat) -> Bus Creator/11  "Xh_sat"
  C_ce/1 -> Bus Creator/12  "C_ce"

== system HORTISIM/Climate/Models/Climate Model/Gases Exchange/Water Dynamics ==
  GasComp : Inport
  Latent Heat : Inport  Port=2
  Condensation : Inport  Port=3
  He : Inport  Port=4
  Te : Inport  Port=5
  Ventilation Rate : Inport  Port=6
  Bus Selector : BusSelector  OutputSignals=QT,Qfog
  Bus Selector1 : BusSelector  OutputSignals=C_w
  Bus Selector2 : BusSelector  OutputSignals=QP_i_c,QP_i_f
  Minus : Sum  Inputs=+-
  Product : Product
  Subsystem : Subsystem
  Vapor Mass Balance : Subsystem
  dC_w_dt : Outport
  wires:
  Ventilation Rate/1 -> Product/1
  Latent Heat/1 -> Bus Selector/1
  Bus Selector/1 -> Vapor Mass Balance/1(<QT_v_i>)  "<QT>"
  GasComp/1 -> Bus Selector1/1
  Bus Selector1/1 -> Minus/1  "<C_w>"
  Condensation/1 -> Bus Selector2/1
  Minus/1 -> Product/2
  Te/1 -> Subsystem/1(<Temperature>)
  He/1 -> Subsystem/2(<Exterior Humidity>)
  Subsystem/1(C_w_Te) -> Minus/2
  Bus Selector/2 -> Vapor Mass Balance/2(<Qfog>)  "<Qfog>"
  Product/1 -> Vapor Mass Balance/3(MW_i_e)
  Bus Selector2/1 -> Vapor Mass Balance/4(<QP_i_c>)  "<QP_i_c>"
  Bus Selector2/2 -> Vapor Mass Balance/5(<QP_i_f>)  "<QP_i_f>"
  Vapor Mass Balance/1(dC_w_dt) -> dC_w_dt/1

== system HORTISIM/Climate/Models/Climate Model/Indoor Temperature Model/Conduction ==
  Indoor Temperature : Inport
  Bus Creator : BusCreator  Inputs=2
  Bus Selector : BusSelector  OutputSignals=Tfloor,Tsoil
  Conduction : MATLAB Function  TreatAsAtomicUnit=on
  Constant : Constant  Value=params.A_f
  Constant1 : Constant  Value=params.lam_s
  Constant2 : Constant  Value=params.l_s
  Constant3 : Constant  Value=params.T_ss
  QD : Outport
  wires:
  Conduction/1(QD_sf1) -> Bus Creator/1
  Conduction/2(QD_s12) -> Bus Creator/2
  Bus Creator/1 -> QD/1
  Indoor Temperature/1 -> Bus Selector/1
  Bus Selector/2 -> Conduction/2(T_s1)  "<Tsoil>"
  Bus Selector/1 -> Conduction/1(T_f)  "<Tfloor>"
  Constant3/1 -> Conduction/6(T_ss)
  Constant2/1 -> Conduction/5(l_s)
  Constant1/1 -> Conduction/4(lam_s)
  Constant/1 -> Conduction/3(A_f)

== system HORTISIM/Climate/Models/Climate Model/Indoor Temperature Model/Convection ==
  In Bus Element2 : Inport  PortName=ExteriorClimate  Element=Temp
  In Bus Element4 : Inport  PortName=ExteriorClimate  Element=Temp
  In Bus Element1 : Inport  PortName=ExteriorClimate  Element=Wind
  In Bus Element3 : Inport  PortName=ExteriorClimate  Element=Wind
  Windows : Inport  Port=2
  Indoor Temperature : Inport  Port=3
  QV_i : Inport  Port=4
  In Bus Element : Inport  Port=5  PortName=Gas  Element=rho_i
  In Bus Element5 : Inport  Port=5  PortName=Gas  Element=C_w
  In Bus Element6 : Inport  Port=5  PortName=Gas  Element=C_w_sat_T_c
  In Bus Element7 : Inport  Port=5  PortName=Gas  Element=C_w_sat_T_f
  Bus Creator : BusCreator  Inputs=5
  Bus Selector1 : BusSelector  OutputSignals=Tair
  Convection : Subsystem
      settings: PortSchema="{\"entries\":[{\"content\":{\"sides\":[{\"content\":{\"connectorIds\":[\"In1\",\"In2\",\"In3\",\"In4\",\"In5\"]},\"type\":\"ConnectorPlacement.EquallySpacedRectSide\",\"uuid\":\"490685c0-4e11-426f-bb8f-3f4d655c5ac7\"},{\"content\":{\"connectorIds\":[\"Out1\",\"Out2\",\"Out3\"],\"side\":\"RIGHT\"},\"type\":\"ConnectorPlacement.EquallySpacedRectSide\",\"uuid\":\"d4812e49-5d44-4dbe-a973-0d0765960a30\"},{\"content\":{\"connectorIds\":[\"In6\",\"In7\"],\"side\":\"TOP\"},\"type\":\"ConnectorPlacement.EquallySpacedRectSide\",\"uuid\":\"13a56147-4397-4d7e-8a08-f4127ff1f422\"},{\"content\":{\"connectorIds\":[\"Out4\"],\"side\":\"BOTTOM\"},\"type\":\"ConnectorPlacement.EquallySpacedRectSide\",\"uuid\":\"3700cf61-bbb7-4a7e-bcc8-2fc27ab64caf\"}]},\"type\":\"ConnectorPlacement.EquallySpacedConnector\",\"uuid\":\"ceadb976-1cc2-4430-962a-7e8db98fda5f\"}],\"packageUris\":[\"http://schema.mathworks.com/mf0/Connector/R2020b\"],\"version\":\"1.0\"}"
  Subsystem : Subsystem
      settings: PortSchema="{\"entries\":[{\"content\":{\"sides\":[{\"content\":{\"connectorIds\":[\"In1\",\"In2\",\"In3\",\"In4\"]},\"type\":\"ConnectorPlacement.EquallySpacedRectSide\",\"uuid\":\"b628b76c-815c-4d2d-bf8b-9241abf78a18\"},{\"content\":{\"connectorIds\":[\"Out1\",\"Out2\"],\"side\":\"RIGHT\"},\"type\":\"ConnectorPlacement.EquallySpacedRectSide\",\"uuid\":\"d01161a9-1f84-445a-b084-f8cb6d6fe506\"},{\"content\":{\"connectorIds\":[],\"side\":\"TOP\"},\"type\":\"ConnectorPlacement.EquallySpacedRectSide\",\"uuid\":\"e7ae8035-b56b-4ea0-80c9-470a91dd5096\"},{\"content\":{\"connectorIds\":[\"In5\"],\"side\":\"BOTTOM\"},\"type\":\"ConnectorPlacement.EquallySpacedRectSide\",\"uuid\":\"28955d4e-ecf1-4383-b712-07fa8a44f693\"}]},\"type\":\"ConnectorPlacement.EquallySpacedConnector\",\"uuid\":\"e2661f4d-c009-47a9-b3ca-7a17d9ffa541\"}],\"packageUris\":[\"http://schema.mathworks.com/mf0/Connector/R2020b\"],\"version\":\"1.0\"}"
  QV : Outport  PortDimensions=5
  QP : Outport  Port=2
  R_a : Outport  Port=3
  wires:
  Indoor Temperature/1 -> Bus Selector1/1, Convection/1(IndoorTemp)
  Convection/4(QP) -> QP/1
  In Bus Element1/1 -> Convection/5(wind_speed)
  In Bus Element4/1 -> Convection/4(T_e)
  In Bus Element5/1 -> Convection/7(C_w)
  In Bus Element/1 -> Subsystem/5(rho_i), Convection/6(rho_i)
  In Bus Element2/1 -> Subsystem/1(T_e)
  In Bus Element3/1 -> Subsystem/2(wind_speed)
  Bus Selector1/1 -> Subsystem/3(<Tair>)  "<Tair>"
  Windows/1 -> Subsystem/4(Windows)
  Subsystem/1(R_a) -> R_a/1
  QV_i/1 -> Bus Creator/5  "QV_i"
  Convection/3(QV_i_f) -> Bus Creator/4
  Convection/2(QV_i_c) -> Bus Creator/3
  Convection/1(QV_c_e) -> Bus Creator/2
  Subsystem/2(QV_i_e) -> Bus Creator/1  "QV_i_e"
  Bus Creator/1 -> QV/1
  In Bus Element6/1 -> Convection/2(Cw_Tc)
  In Bus Element7/1 -> Convection/3(Cw_Tf)

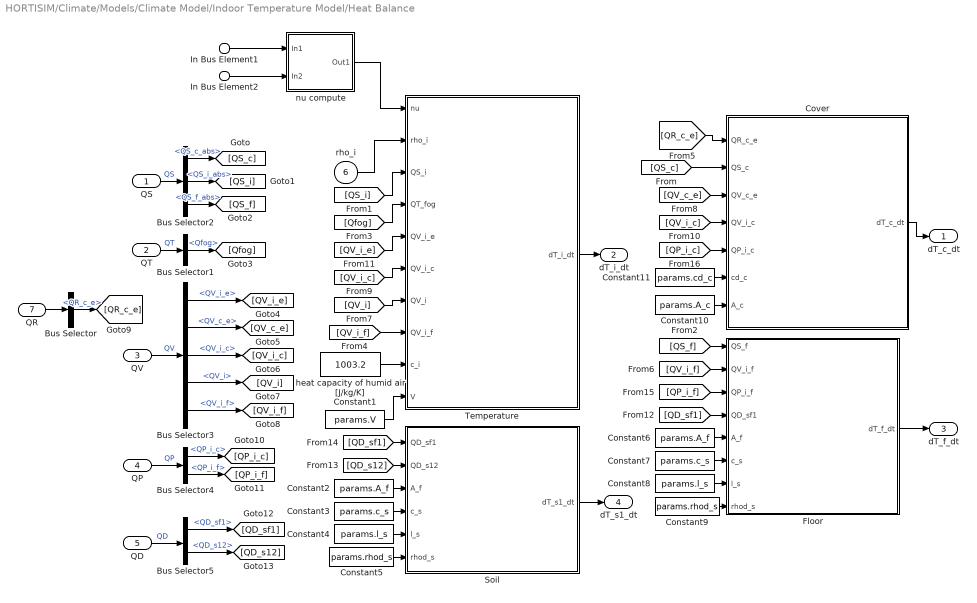
== system HORTISIM/Climate/Models/Climate Model/Indoor Temperature Model/Heat Balance ==
  QS : Inport
  QT : Inport  Port=2
  QV : Inport  Port=3
  QP : Inport  Port=4
  QD : Inport  Port=5
  rho_i : Inport  Port=6
  QR : Inport  Port=7
  In Bus Element1 : Inport  Port=8  PortName=screen  Element=beta
  In Bus Element2 : Inport  Port=8  PortName=screen  Element=value
  " Cover" : MATLAB Function  TreatAsAtomicUnit=on
  " Floor" : MATLAB Function  TreatAsAtomicUnit=on
  " Soil" : MATLAB Function  TreatAsAtomicUnit=on
  " Temperature" : MATLAB Function  TreatAsAtomicUnit=on
  Bus Selector : BusSelector  OutputSignals=QR_c_e
  Bus Selector1 : BusSelector  OutputSignals=Qfog
  Bus Selector2 : BusSelector  OutputSignals=QS_c_abs,QS_i_abs,QS_f_abs
  Bus Selector3 : BusSelector  OutputSignals=QV_i_e,QV_c_e,QV_i_c,QV_i,QV_i_f
  Bus Selector4 : BusSelector  OutputSignals=QP_i_c,QP_i_f
  Bus Selector5 : BusSelector  OutputSignals=QD_sf1,QD_s12
  Constant1 : Constant  Value=params.V
  Constant10 : Constant  Value=params.A_c
  Constant11 : Constant  Value=params.cd_c
  Constant2 : Constant  Value=params.A_f
  Constant3 : Constant  Value=params.c_s
  Constant4 : Constant  Value=params.l_s
  Constant5 : Constant  Value=params.rhod_s
  Constant6 : Constant  Value=params.A_f
  Constant7 : Constant  Value=params.c_s
  Constant8 : Constant  Value=params.l_s
  Constant9 : Constant  Value=params.rhod_s
  "heat capacity of humid air [J/kg/K] " : Constant  Value=1003.2
  nu compute : Subsystem
  dT_c_dt : Outport
  dT_i_dt : Outport  Port=2
  dT_f_dt : Outport  Port=3
  dT_s1_dt : Outport  Port=4
  wires:
  nu compute/1(Out1) -> " Temperature"/1(nu)
  In Bus Element2/1 -> nu compute/2(In2)
  In Bus Element1/1 -> nu compute/1(In1)
  " Floor"/1(dT_f_dt) -> dT_f_dt/1
  " Soil"/1(dT_s1_dt) -> dT_s1_dt/1
  QD/1 -> Bus Selector5/1  "QD"
  " Temperature"/1(dT_i_dt) -> dT_i_dt/1
  QT/1 -> Bus Selector1/1  "QT"
  QS/1 -> Bus Selector2/1  "QS"
  QP/1 -> Bus Selector4/1  "QP"
  rho_i/1 -> " Temperature"/2(rho_i)
  QV/1 -> Bus Selector3/1  "QV"
  " Cover"/1(dT_c_dt) -> dT_c_dt/1
  Bus Selector2/1 -> [QS_c]  "<QS_c_abs>"
  Bus Selector2/2 -> [QS_i]  "<QS_i_abs>"
  Bus Selector2/3 -> [QS_f]  "<QS_f_abs>"
  [QS_c] -> " Cover"/2(QS_c)
  [QS_i] -> " Temperature"/3(QS_i)
  [QS_f] -> " Floor"/1(QS_f)
  Bus Selector1/1 -> [Qfog]  "<Qfog>"
  [Qfog] -> " Temperature"/4(QT_fog)
  Bus Selector3/1 -> [QV_i_e]  "<QV_i_e>"
  Bus Selector3/5 -> [QV_i_f]  "<QV_i_f>"
  Bus Selector3/4 -> [QV_i]  "<QV_i>"
  Bus Selector3/3 -> [QV_i_c]  "<QV_i_c>"
  Bus Selector3/2 -> [QV_c_e]  "<QV_c_e>"
  [QV_i_f] -> " Temperature"/8(QV_i_f)
  [QV_i_f] -> " Floor"/2(QV_i_f)
  [QV_i] -> " Temperature"/7(QV_i)
  [QV_c_e] -> " Cover"/3(QV_c_e)
  [QV_i_c] -> " Temperature"/6(QV_i_c)
  [QV_i_c] -> " Cover"/4(QV_i_c)
  [QV_i_e] -> " Temperature"/5(QV_i_e)
  Bus Selector4/1 -> [QP_i_c]  "<QP_i_c>"
  Bus Selector4/2 -> [QP_i_f]  "<QP_i_f>"
  Bus Selector5/1 -> [QD_sf1]  "<QD_sf1>"
  Bus Selector5/2 -> [QD_s12]  "<QD_s12>"
  [QD_sf1] -> " Floor"/4(QD_sf1)
  [QD_s12] -> " Soil"/2(QD_s12)
  [QD_sf1] -> " Soil"/1(QD_sf1)
  [QP_i_f] -> " Floor"/3(QP_i_f)
  [QP_i_c] -> " Cover"/5(QP_i_c)
  "heat capacity of humid air [J/kg/K] "/1 -> " Temperature"/9(c_i)
  Constant1/1 -> " Temperature"/10(V)
  Constant2/1 -> " Soil"/3(A_f)
  Constant3/1 -> " Soil"/4(c_s)
  Constant4/1 -> " Soil"/5(l_s)
  Constant5/1 -> " Soil"/6(rhod_s)
  Constant6/1 -> " Floor"/5(A_f)
  Constant7/1 -> " Floor"/6(c_s)
  Constant8/1 -> " Floor"/7(l_s)
  Constant9/1 -> " Floor"/8(rhod_s)
  Constant10/1 -> " Cover"/7(A_c)
  Constant11/1 -> " Cover"/6(cd_c)
  QR/1 -> Bus Selector/1
  Bus Selector/1 -> [QR_c_e]  "<QR_c_e>"
  [QR_c_e] -> " Cover"/1(QR_c_e)
